simulink model "untitled"  (R2017b)
settings: Solver=FixedStepAuto  StartTime=0.0  StopTime=0.08  FixedStep=5e-6  RelTol=1e-3
undefined symbols (not defined in the file): fdesignblkfcn, gcbh
libraries: simulink x1, dspfdesign x1, dsparch4 x1, powerlib x1
(part 1 of 3)
settings Model: Creator=zsrx  LastModifiedBy=zsrx

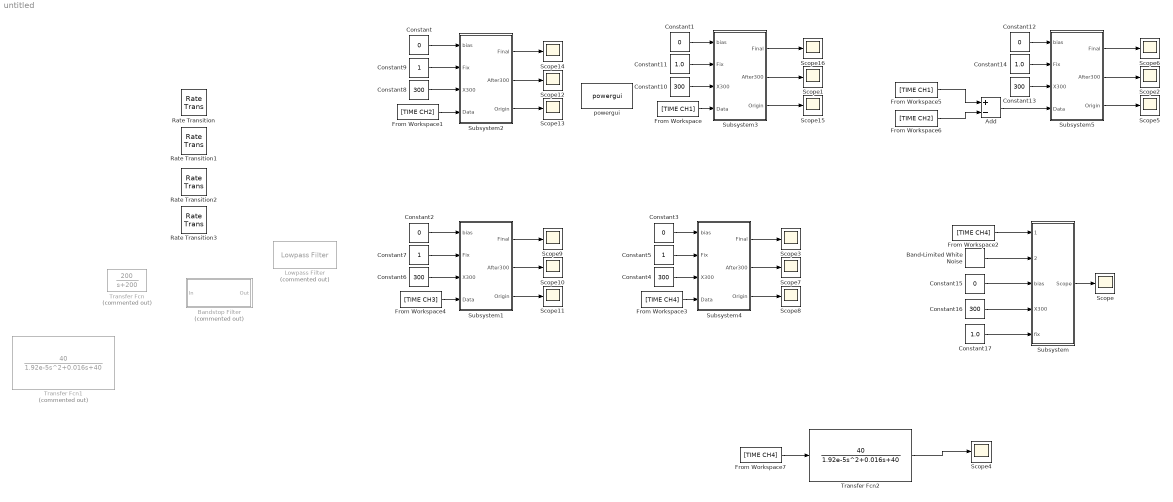
== system untitled ==
  Add : Sum  Inputs=+-
  Band-Limited White Noise : simulink/Sources/Band-Limited White Noise  Cov=[0.0000000001]  Ts=5e-6  seed=[23341]
  Bandstop Filter : Subsystem  Commented=on  DialogController=fdesignblkfcn  InitFcn=fdesignblkfcn(gcbh, {'InitFcn'});  mask(Bandstop Filter){}
      mask help: Design a bandstop filter
      settings: CopyFcn=fdesignblkfcn(gcbh, {'CopyFcn'});
      mask Help: helpview(mapfilelocation('dsp'), 'dspbandstopfilter');
      mask Display: disp('Bandstop');
  Constant{,1..3,12,15} (6 alike) : Constant  Value=0
  Constant{4,6,8,10,13,16} (6 alike) : Constant  Value=300
  Constant11 : Constant  Value=1.0
  Constant14 : Constant  Value=1.0
  Constant17 : Constant  Value=1.0
  Constant5 : Constant
  Constant7 : Constant
  Constant9 : Constant
  From Workspace : FromWorkspace  VariableName=[TIME CH1]  SampleTime=0
  From Workspace1 : FromWorkspace  VariableName=[TIME CH2]  SampleTime=0
  From Workspace2 : FromWorkspace  VariableName=[TIME CH4]  SampleTime=0
  From Workspace3 : FromWorkspace  VariableName=[TIME CH4]  SampleTime=0
  From Workspace4 : FromWorkspace  VariableName=[TIME CH3]  SampleTime=0
  From Workspace5 : FromWorkspace  VariableName=[TIME CH1]  SampleTime=0
  From Workspace6 : FromWorkspace  VariableName=[TIME CH2]  SampleTime=0
  From Workspace7 : FromWorkspace  VariableName=[TIME CH4]  SampleTime=0
  Lowpass Filter : dspfdesign/Lowpass Filter  Commented=on  FilterType=FIR  DesignForMinimumOrder=on  FilterOrder=50  PassbandFrequency=400  StopbandFrequency=500  PassbandRipple=0.1  StopbandAttenuation=80  InheritSampleRate=off  SampleRate=44100  SimulateUsing=Interpreted execution  roundingMode=Floor  coeffsDataTypeStr=fixdt(1,16)
  Rate Transition{,1..3} (4 alike) : RateTransition  OutPortSampleTime=5e-5
  Scope{,1..16} (17 alike) : Scope
  Subsystem : Subsystem
  Subsystem1 : Subsystem
  Subsystem2 : Subsystem
  Subsystem3 : Subsystem
  Subsystem4 : Subsystem
  Subsystem5 : Subsystem
  Transfer Fcn : TransferFcn  Commented=on  Numerator=[200]  Denominator=[1 200]
  Transfer Fcn1 : TransferFcn  Commented=on  Numerator=[40]  Denominator=[1.92e-5 0.016 40]
  Transfer Fcn2 : TransferFcn  Numerator=[40]  Denominator=[1.92e-5 0.016 40]
  powergui : powerlib/powergui  Priority=1  SimulationMode=Discrete  SampleTime=5e-6  frequency=60  Iterations=50  frequencyindice=60  Pbase=100e6  ErrMax=1e-4  UnitsV=kV  UnitsW=MW  buscounter=0  FunctionMessages=off  echomessages=off  EnableUseOfTLC=off  CurrentSourceSwitches=off  DisableSnubberDevices=off  DisableRonSwitches=off  DisableVfSwitches=off  DisplayEquations=off  SolverType=Tustin/Backward Euler (TBE)  Interpol=off  ExternalGateDelay=off  methode=off  Ts=100  x0status=blocks  SPID=off  SwTol=0  HookPort=off  RestoreLinks=warning  ResistiveCurrentMeasurement=off  Frange=[0:2:500]  Ylog=off  Xlog=on  ShowGrid=off  save=off  variable=ZData  structure=ScopeData1  ZoomFFT=off  StartTime=0.02  cycles=1  DisplayStyle=2  fundamental=50  FreqAxis=off  MaxFrequency=10000  frequencyindicesteady=1  RmsSteady=1  display=off
  wires:
  From Workspace3/1 -> Subsystem4/4(Data)
  Subsystem4/1(Final) -> Scope3/1
  Constant4/1 -> Subsystem4/3(X300)
  Constant5/1 -> Subsystem4/2(Fix)
  Subsystem4/2(After300) -> Scope7/1
  Subsystem4/3(Origin) -> Scope8/1
  From Workspace4/1 -> Subsystem1/4(Data)
  Subsystem1/1(Final) -> Scope9/1
  Subsystem1/2(After300) -> Scope10/1
  Subsystem1/3(Origin) -> Scope11/1
  Constant7/1 -> Subsystem1/2(Fix)
  Constant6/1 -> Subsystem1/3(X300)
  Constant9/1 -> Subsystem2/2(Fix)
  Subsystem2/1(Final) -> Scope14/1
  Subsystem2/2(After300) -> Scope12/1
  From Workspace1/1 -> Subsystem2/4(Data)
  Constant8/1 -> Subsystem2/3(X300)
  Subsystem2/3(Origin) -> Scope13/1
  Constant11/1 -> Subsystem3/2(Fix)
  Subsystem3/3(Origin) -> Scope15/1
  Constant10/1 -> Subsystem3/3(X300)
  Subsystem3/2(After300) -> Scope1/1
  Subsystem3/1(Final) -> Scope16/1
  Constant/1 -> Subsystem2/1(bias)
  From Workspace/1 -> Subsystem3/4(Data)
  Constant1/1 -> Subsystem3/1(bias)
  Constant2/1 -> Subsystem1/1(bias)
  Constant3/1 -> Subsystem4/1(bias)
  From Workspace2/1 -> Subsystem/1(Source)
  Band-Limited White Noise/1 -> Subsystem/2(Random)
  Subsystem/1(Scope) -> Scope/1
  From Workspace5/1 -> Add/1
  From Workspace6/1 -> Add/2
  Add/1 -> Subsystem5/4(Data)
  Constant13/1 -> Subsystem5/3(X300)
  Constant14/1 -> Subsystem5/2(Fix)
  Constant12/1 -> Subsystem5/1(bias)
  Subsystem5/3(Origin) -> Scope5/1
  Subsystem5/2(After300) -> Scope2/1
  Subsystem5/1(Final) -> Scope6/1
  Constant15/1 -> Subsystem/3(bias)
  Constant16/1 -> Subsystem/4(X300)
  Constant17/1 -> Subsystem/5(fix)
  From Workspace7/1 -> Transfer Fcn2/1
  Transfer Fcn2/1 -> Scope4/1
